simulink model "minesweeper_stateflow"  (R2024a)
settings: Solver=FixedStepDiscrete  StartTime=0.0  StopTime=120  FixedStep=0.1  RelTol=1e-3
settings Model: Creator=yousef  LastModifiedBy=yousef

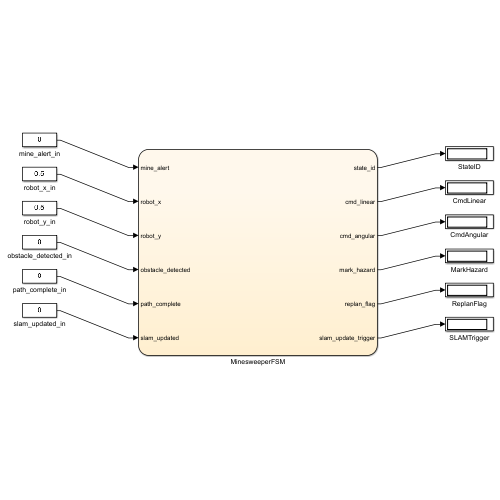
[thumbnail: Simulink's stored preview of the top-level diagram]
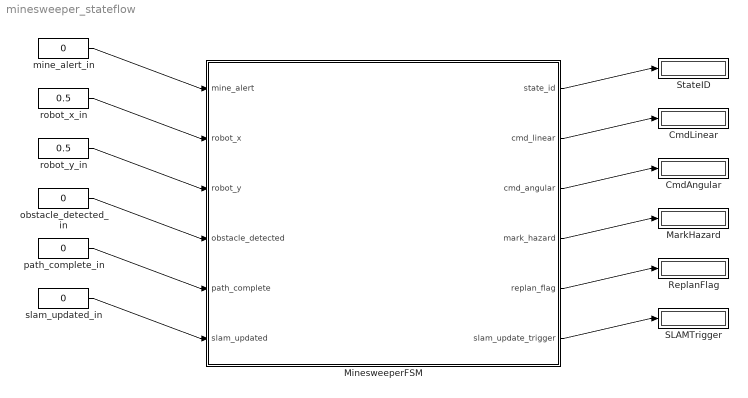
== system minesweeper_stateflow ==
  CmdAngular : Display
  CmdLinear : Display
  MarkHazard : Display
  MinesweeperFSM : Stateflow chart  TreatAsAtomicUnit=on
  ReplanFlag : Display
  SLAMTrigger : Display
  StateID : Display
  mine_alert_in : Constant  Value=0
  obstacle_detected_in : Constant  Value=0
  path_complete_in : Constant  Value=0
  robot_x_in : Constant  Value=0.5
  robot_y_in : Constant  Value=0.5
  slam_updated_in : Constant  Value=0
  wires:
  mine_alert_in/1 -> MinesweeperFSM/1(mine_alert)
  robot_x_in/1 -> MinesweeperFSM/2(robot_x)
  robot_y_in/1 -> MinesweeperFSM/3(robot_y)
  obstacle_detected_in/1 -> MinesweeperFSM/4(obstacle_detected)
  path_complete_in/1 -> MinesweeperFSM/5(path_complete)
  slam_updated_in/1 -> MinesweeperFSM/6(slam_updated)
  MinesweeperFSM/1(state_id) -> StateID/1
  MinesweeperFSM/2(cmd_linear) -> CmdLinear/1
  MinesweeperFSM/3(cmd_angular) -> CmdAngular/1
  MinesweeperFSM/4(mark_hazard) -> MarkHazard/1
  MinesweeperFSM/5(replan_flag) -> ReplanFlag/1
  MinesweeperFSM/6(slam_update_trigger) -> SLAMTrigger/1

== stateflow chart minesweeper_stateflow/MinesweeperFSM ==
  state Explore
    entry: state_id=1; cmd_linear=0.5; cmd_angular=0;
    mark_hazard=0; replan_flag=0;
    during: distance=robot_x+robot_y;
  state DetectObstacle
    entry: state_id=2; cmd_linear=0;
    obstacle_x=robot_x; obstacle_y=robot_y;
    known_obstacles=known_obstacles+1;
  state ReplanPath
    entry: state_id=4; replan_flag=1; cmd_linear=0;
    during: distance=abs(robot_x-obstacle_x)+abs(robot_y-obstacle_y);
  state UpdateSLAM
    entry: state_id=3; slam_update_trigger=1;
    during: if slam_updated==1, slam_update_trigger=0; end
  state DetectMine
    entry: state_id=5; cmd_linear=0; mark_hazard=1;
    mine_x=robot_x; mine_y=robot_y;
    known_mines=known_mines+1;
  state MissionComplete
    entry: state_id=6; cmd_linear=0; cmd_angular=0;
    replan_flag=0; mark_hazard=0;
  (default) -> Explore
  ReplanPath -> Explore : after(0.5,sec)
  Explore -> DetectObstacle [order 1] : [obstacle_detected==1]
  UpdateSLAM -> ReplanPath : after(0.3,sec)
  Explore -> MissionComplete [order 3] : [path_complete==1]
  DetectObstacle -> UpdateSLAM : after(0.2,sec)
  Explore -> DetectMine [order 2] : [mine_alert==1]
  DetectMine -> UpdateSLAM : after(0.5,sec)
  data: mine_alert input; robot_x input; robot_y input; obstacle_detected input; path_complete input; slam_updated input; state_id output; cmd_linear output; cmd_angular output; mark_hazard output; replan_flag output; slam_update_trigger output; obstacle_x local; obstacle_y local; mine_x local; mine_y local; distance local; known_obstacles local; known_mines local
